simulink subsystem "s3s_to_2e"  (R2022b)
settings: Solver=VariableStepAuto  StartTime=0.0  StopTime=10.0  RelTol=1e-3
settings Model: Creator=jack  LastModifiedBy=jack

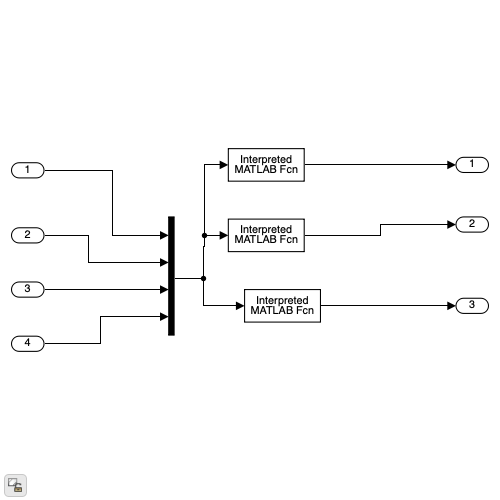
[thumbnail: Simulink's stored preview of the top-level diagram]
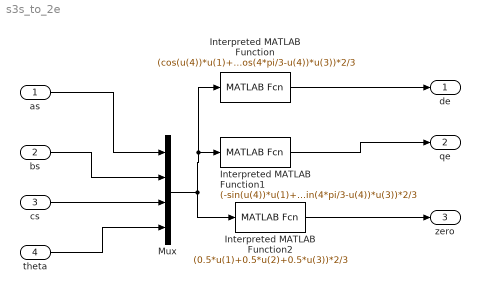
== system s3s_to_2e ==
  as : Inport
  bs : Inport  Port=2
  cs : Inport  Port=3
  theta : Inport  Port=4
  Interpreted MATLAB Function : MATLABFcn  MATLABFcn=(cos(u(4))*u(1)+cos(2*pi/3-u(4))*u(2)+cos(4*pi/3-u(4))*u(3))*2/3
  Interpreted MATLAB Function1 : MATLABFcn  MATLABFcn=(-sin(u(4))*u(1)+sin(2*pi/3-u(4))*u(2)+sin(4*pi/3-u(4))*u(3))*2/3
  Interpreted MATLAB Function2 : MATLABFcn  MATLABFcn=(0.5*u(1)+0.5*u(2)+0.5*u(3))*2/3
  Mux : Mux
  de : Outport
  qe : Outport  Port=2
  zero : Outport  Port=3
  wires:
  bs/1 -> Mux/2
  cs/1 -> Mux/3
  Interpreted MATLAB Function/1 -> de/1
  theta/1 -> Mux/4
  Interpreted MATLAB Function2/1 -> zero/1
  Mux/1 -> Interpreted MATLAB Function2/1, Interpreted MATLAB Function1/1, Interpreted MATLAB Function/1
  Interpreted MATLAB Function1/1 -> qe/1
  as/1 -> Mux/1
